simulink model "laba1"  (R2022a)
settings: Solver=FixedStepAuto  StartTime=0.0  StopTime=1e6  RelTol=1e-3
settings Model: Creator=User  LastModifiedBy=User

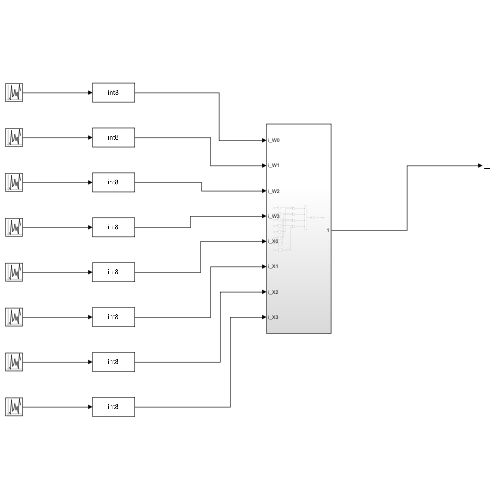
[thumbnail: Simulink's stored preview of the top-level diagram]
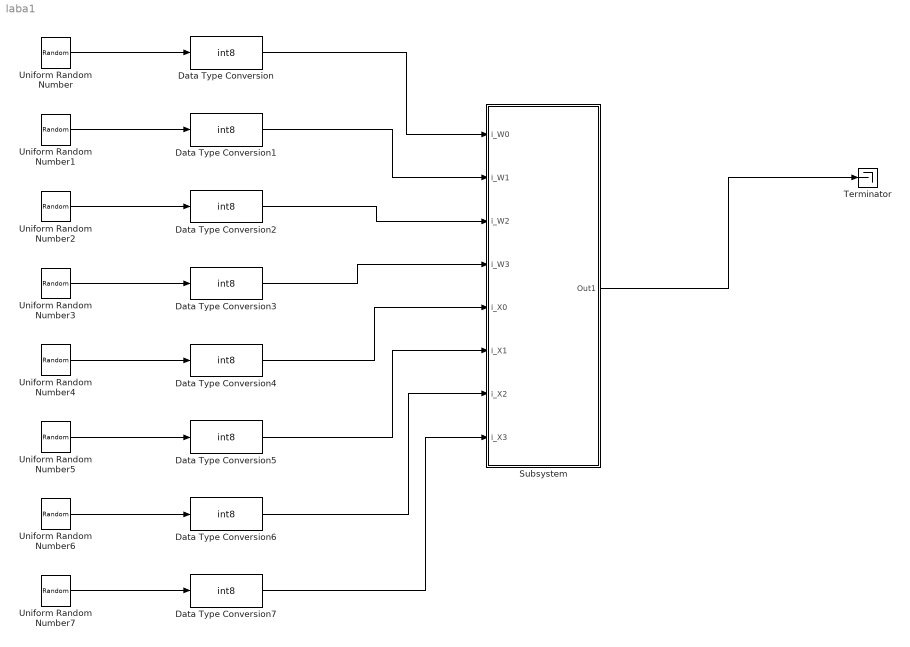
== system laba1 ==
  Data Type Conversion{,1..7} (8 alike) : DataTypeConversion  OutDataTypeStr=int8  SaturateOnIntegerOverflow=off  RndMeth=Floor  LockScale=on
  Subsystem : Subsystem
  Terminator : Terminator
  Uniform Random Number : UniformRandomNumber  Minimum=0  Maximum=2^8-1  Seed=14  SampleTime=1
  Uniform Random Number1 : UniformRandomNumber  Minimum=0  Maximum=2^8-1  Seed=15  SampleTime=1
  Uniform Random Number2 : UniformRandomNumber  Minimum=0  Maximum=2^8-1  Seed=16  SampleTime=1
  Uniform Random Number3 : UniformRandomNumber  Minimum=0  Maximum=2^8-1  Seed=17  SampleTime=1
  Uniform Random Number4 : UniformRandomNumber  Minimum=0  Maximum=2^8-1  Seed=18  SampleTime=1
  Uniform Random Number5 : UniformRandomNumber  Minimum=0  Maximum=2^8-1  Seed=19  SampleTime=1
  Uniform Random Number6 : UniformRandomNumber  Minimum=0  Maximum=2^8-1  Seed=20  SampleTime=1
  Uniform Random Number7 : UniformRandomNumber  Minimum=0  Maximum=2^8-1  Seed=21  SampleTime=1
  wires:
  Uniform Random Number/1 -> Data Type Conversion/1
  Uniform Random Number1/1 -> Data Type Conversion1/1
  Uniform Random Number2/1 -> Data Type Conversion2/1
  Uniform Random Number3/1 -> Data Type Conversion3/1
  Uniform Random Number4/1 -> Data Type Conversion4/1
  Uniform Random Number5/1 -> Data Type Conversion5/1
  Uniform Random Number6/1 -> Data Type Conversion6/1
  Uniform Random Number7/1 -> Data Type Conversion7/1
  Data Type Conversion/1 -> Subsystem/1(i_W0)
  Data Type Conversion1/1 -> Subsystem/2(i_W1)
  Data Type Conversion2/1 -> Subsystem/3(i_W2)
  Data Type Conversion3/1 -> Subsystem/4(i_W3)
  Data Type Conversion4/1 -> Subsystem/5(i_X0)
  Data Type Conversion5/1 -> Subsystem/6(i_X1)
  Data Type Conversion6/1 -> Subsystem/7(i_X2)
  Data Type Conversion7/1 -> Subsystem/8(i_X3)
  Subsystem/1(Out1) -> Terminator/1

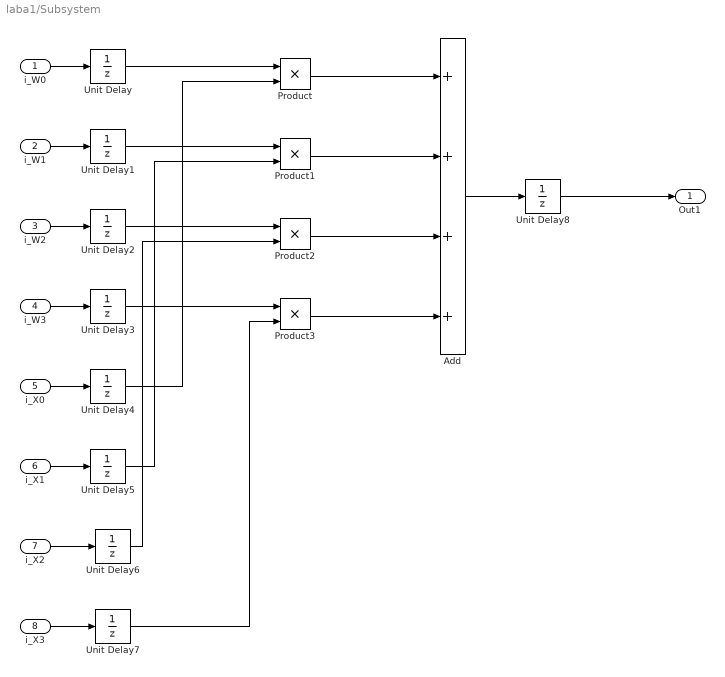
== system laba1/Subsystem ==
  i_W0 : Inport
  i_W1 : Inport  Port=2
  i_W2 : Inport  Port=3
  i_W3 : Inport  Port=4
  i_X0 : Inport  Port=5
  i_X1 : Inport  Port=6
  i_X2 : Inport  Port=7
  i_X3 : Inport  Port=8
  Add : Sum  Inputs=++++
  Product{,1..3} (4 alike) : Product
  Unit Delay{,1..8} (9 alike) : UnitDelay  SampleTime=-1  HasFrameUpgradeWarning=on
  Out1 : Outport
  wires:
  Product3/1 -> Add/4
  Product/1 -> Add/1
  Product2/1 -> Add/3
  i_W0/1 -> Unit Delay/1
  Product1/1 -> Add/2
  i_W1/1 -> Unit Delay1/1
  i_W3/1 -> Unit Delay3/1
  i_W2/1 -> Unit Delay2/1
  i_X0/1 -> Unit Delay4/1
  i_X2/1 -> Unit Delay6/1
  i_X3/1 -> Unit Delay7/1
  Unit Delay/1 -> Product/1
  Unit Delay1/1 -> Product1/1
  Unit Delay2/1 -> Product2/1
  Unit Delay3/1 -> Product3/1
  Unit Delay4/1 -> Product/2
  Unit Delay5/1 -> Product1/2
  Unit Delay6/1 -> Product2/2
  Unit Delay7/1 -> Product3/2
  i_X1/1 -> Unit Delay5/1
  Add/1 -> Unit Delay8/1
  Unit Delay8/1 -> Out1/1
